simulink model "Actuator_Control"  (R2014b)
settings: Solver=FixedStepDiscrete  StartTime=0.0  StopTime=inf  FixedStep=sample_time  RelTol=1e-3
undefined symbols (not defined in the file): A1_notch_f1, A2_notch_f1, A_lpf_accel, A_lpf_dtau, B1_lpf_accel, B1_lpf_dtau, B1_notch_f1, B2_lpf_accel, B2_lpf_dtau, B2_notch_f1, gain_nodes_sea_torque, j_motor, j_segments, k_ff, K_notch_f1, k_sea, kd_loaded_sea, kd_sea_torque, kd_sea_torque_flight, kd_sea_torque_stance, kp_loaded_sea, kp_sea_torque, kp_sea_torque_flight, kp_sea_torque_stance, loaded_unloaded_sigmoid_width, loaded_unloaded_torque_threshold, max_sagittal_loaded_torque, max_sagittal_unloaded_torque, sample_time, sea_control_torque_cmd_small_threshold, sea_coulomb_friction, sea_coulomb_friction_direction_switch_sensitivity, sea_extra_sliding_friction, sea_offset_friction, stance_flight_torque_threshold
libraries: simulink x8
settings Model: BufferReuse=off  Creator=wmartin  LastModifiedBy=wmartin
settings SolverCC: EnableConcurrentExecution=on
settings DataIOCC: MaxDataPoints=1000000000  SaveFormat=StructureWithTime  SaveOutput=off  SaveTime=off
settings OptimizationCC: BlockReduction=off  OptimizeBlockIOStorage=off  BufferReuse=off  GlobalBufferReuse=off  ExpressionFolding=off  LocalBlockOutputs=off  SimCompilerOptimization=On
settings HardwareCC: ProdIntDivRoundTo=Zero  ProdEndianess=LittleEndian  ProdLongLongMode=on  ProdHWDeviceType=Generic->32-bit x86 compatible
settings ModelReferenceCC: UpdateModelReferenceTargets=AssumeUpToDate  ModelReferenceNumInstancesAllowed=Single  ModelReferenceMinAlgLoopOccurrences=on
settings RTWCC: SystemTargetFile=slrt.tlc  TemplateMakefile=slrt_default_tmf  Description=Simulink Real-Time  RTWVerbose=off  ProcessScript=slrt_make_rtw_hook  RTWCompilerOptimization=On
settings SimulinkRealTimeCC: GeneratePreprocessorConditionals=Disable all  EnableShiftOperators=on  RL32LogBufSizeModifier=100000000

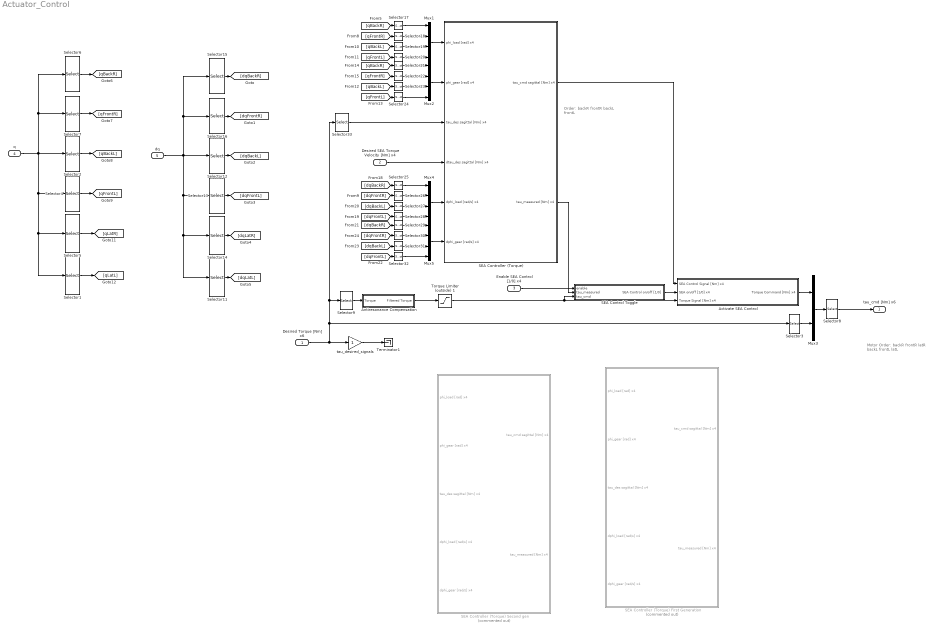
== system Actuator_Control ==
  note: Order:
      | backR
      | frontR
      | backL
      | frontL
  note: Motor Order:
      |
      | backR
      | frontR
      | latR
      | backL
      | frontL
      | latL
  Desired Torque [Nm] x6 : Inport  OutDataTypeStr=double  PortDimensions=6  SampleTime=sample_time
  Desired SEA Torque Velocity [Nm] x4 : Inport  Port=2  OutDataTypeStr=double  PortDimensions=4  SampleTime=sample_time
  Enable SEA Control [1/0] x4 : Inport  Port=3  OutDataTypeStr=boolean  PortDimensions=4  SampleTime=sample_time
  q : Inport  Port=4  OutDataTypeStr=double  PortDimensions=13  SampleTime=sample_time
  dq : Inport  Port=5  OutDataTypeStr=double  PortDimensions=13  SampleTime=sample_time
  Activate SEA Control : Subsystem
  Antiresonance Compensation : Subsystem
  Mux{1..2,4..5} (4 alike) : Mux
  Mux3 : Mux  Inputs=2
  SEA Control Toggle : Subsystem
  SEA Controller (Torque) : Subsystem
  SEA Controller (Torque) First Generation : Subsystem  Commented=on
  SEA Controller (Torque) Second gen : Subsystem  Commented=on
  Selector1 : Selector  InputPortWidth=13  Indices=[10]
  Selector11 : Selector  InputPortWidth=13  Indices=[10]
  Selector12 : Selector  InputPortWidth=13  Indices=[5 6]
  Selector13 : Selector  InputPortWidth=13  Indices=[7 8]
  Selector14 : Selector  InputPortWidth=13  Indices=[9]
  Selector15 : Selector  InputPortWidth=13  Indices=[1 2]
  Selector16 : Selector  InputPortWidth=13  Indices=[3 4]
  Selector{17..20,25..28} (8 alike) : Selector  InputPortWidth=2  Indices=[1]
  Selector2 : Selector  InputPortWidth=13  Indices=[5 6]
  Selector{21..24,29..32} (8 alike) : Selector  InputPortWidth=2  Indices=[2]
  Selector3 : Selector  InputPortWidth=6  Indices=[3 6]
  Selector33 : Selector  InputPortWidth=6  Indices=[1 2 4 5]
  Selector4 : Selector  InputPortWidth=13  Indices=[7 8]
  Selector5 : Selector  InputPortWidth=13  Indices=[9]
  Selector6 : Selector  InputPortWidth=13  Indices=[1 2]
  Selector7 : Selector  InputPortWidth=13  Indices=[3 4]
  Selector8 : Selector  InputPortWidth=6  Indices=[1 2 5 3 4 6]
  Selector9 : Selector  InputPortWidth=6  Indices=[1 2 4 5]
  Terminator1 : Terminator
  Torque Limiter (outside) 1 : Saturate  UpperLimit=max_sagittal_unloaded_torque  LowerLimit=-max_sagittal_unloaded_torque
      settings: AttributesFormatString=Hi: %<UpperLimit>\nLo: %<LowerLimit>
  tau_desired_signals : Gain  Description=xPCTag(1)=tau_cmd_signal;
  tau_cmd [Nm] x6 : Outport  OutDataTypeStr=double  PortDimensions=6  SampleTime=0  InitialOutput=[0 0 0 0 0 0]
  wires:
  Selector9/1 -> Antiresonance Compensation/1(Torque)
  SEA Controller (Torque)/2(tau_measured [Nm] x4) -> SEA Control Toggle/2(tau_measured)
  SEA Controller (Torque)/1(tau_cmd sagittal [Nm] x4) -> Activate SEA Control/1(SEA Control Signal [Nm] x4)
  Torque Limiter (outside) 1/1 -> Activate SEA Control/3(Torque Signal [Nm] x4), SEA Control Toggle/3(tau_cmd)
  Activate SEA Control/1(Torque Command [Nm] x4) -> Mux3/1
  Desired Torque [Nm] x6/1 -> Selector33/1, Selector9/1, Selector3/1, tau_desired_signals/1
  Selector8/1 -> tau_cmd [Nm] x6/1
  tau_desired_signals/1 -> Terminator1/1
  Selector5/1 -> [qLatR]
  Selector1/1 -> [qLatL]
  Selector6/1 -> [qBackR]
  Selector7/1 -> [qFrontR]
  Selector2/1 -> [qBackL]
  Selector4/1 -> [qFrontL]
  q/1 -> Selector2/1, Selector7/1, Selector6/1, Selector4/1, Selector5/1, Selector1/1
  dq/1 -> Selector11/1, Selector14/1, Selector13/1, Selector15/1, Selector16/1, Selector12/1
  Selector14/1 -> [dqLatR]
  Selector11/1 -> [dqLatL]
  Selector15/1 -> [dqBackR]
  Selector16/1 -> [dqFrontR]
  Selector12/1 -> [dqBackL]
  Selector13/1 -> [dqFrontL]
  Mux1/1 -> SEA Controller (Torque)/1(phi_load [rad] x4)
  [qBackR] -> Selector17/1
  Selector17/1 -> Mux1/1
  Selector19/1 -> Mux1/3
  Selector18/1 -> Mux1/2
  Selector20/1 -> Mux1/4
  [qFrontR] -> Selector18/1
  [qBackL] -> Selector19/1
  [qFrontL] -> Selector20/1
  Mux2/1 -> SEA Controller (Torque)/2(phi_gear [rad] x4)
  [qBackR] -> Selector21/1
  Selector21/1 -> Mux2/1
  Selector23/1 -> Mux2/3
  Selector22/1 -> Mux2/2
  Selector24/1 -> Mux2/4
  [qFrontR] -> Selector22/1
  [qBackL] -> Selector23/1
  [qFrontL] -> Selector24/1
  Mux4/1 -> SEA Controller (Torque)/5(dphi_load [rad/s] x4)
  [dqBackR] -> Selector25/1
  Selector25/1 -> Mux4/1
  Selector27/1 -> Mux4/3
  Selector26/1 -> Mux4/2
  Selector28/1 -> Mux4/4
  [dqFrontR] -> Selector26/1
  [dqBackL] -> Selector27/1
  [dqFrontL] -> Selector28/1
  Mux5/1 -> SEA Controller (Torque)/6(dphi_gear [rad/s] x4)
  [dqBackR] -> Selector29/1
  Selector29/1 -> Mux5/1
  Selector31/1 -> Mux5/3
  Selector30/1 -> Mux5/2
  Selector32/1 -> Mux5/4
  [dqFrontR] -> Selector30/1
  [dqBackL] -> Selector31/1
  [dqFrontL] -> Selector32/1
  Selector33/1 -> SEA Controller (Torque)/3(tau_des sagittal [Nm] x4)
  Selector3/1 -> Mux3/2
  Mux3/1 -> Selector8/1
  Enable SEA Control [1/0] x4/1 -> SEA Control Toggle/1(enable)
  Antiresonance Compensation/1(Filtered Torque) -> Torque Limiter (outside) 1/1
  SEA Control Toggle/1(SEA Control on/off [1/0]) -> Activate SEA Control/2("SEA on/off [1/0] x4 ")
  Desired SEA Torque Velocity [Nm] x4/1 -> SEA Controller (Torque)/4(dtau_des sagittal [Nm] x4)

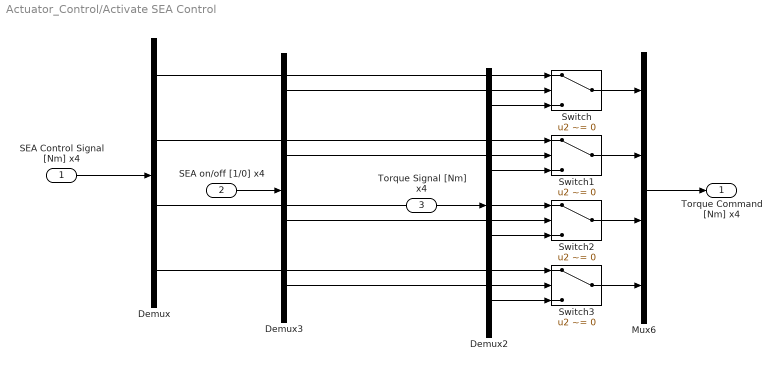
== system Actuator_Control/Activate SEA Control ==
  SEA Control Signal [Nm] x4 : Inport
  "SEA on/off [1/0] x4 " : Inport  Port=2
  Torque Signal [Nm] x4 : Inport  Port=3
  Demux : Demux
  Demux2 : Demux
  Demux3 : Demux
  Mux6 : Mux
  Switch{,1..3} (4 alike) : Switch  Criteria=u2 ~= 0
  Torque Command [Nm] x4 : Outport
  wires:
  Demux2/2 -> Switch1/3
  Demux2/1 -> Switch/3
  Demux/1 -> Switch/1
  Switch/1 -> Mux6/1
  Switch1/1 -> Mux6/2
  Switch3/1 -> Mux6/4
  Demux3/1 -> Switch/2
  Mux6/1 -> Torque Command [Nm] x4/1
  Demux3/3 -> Switch2/2
  Demux3/2 -> Switch1/2
  Demux/3 -> Switch2/1
  Switch2/1 -> Mux6/3
  Demux/4 -> Switch3/1
  Demux2/4 -> Switch3/3
  Demux3/4 -> Switch3/2
  Demux/2 -> Switch1/1
  Demux2/3 -> Switch2/3
  SEA Control Signal [Nm] x4/1 -> Demux/1
  "SEA on/off [1/0] x4 "/1 -> Demux3/1
  Torque Signal [Nm] x4/1 -> Demux2/1

== system Actuator_Control/Antiresonance Compensation ==
  Torque : Inport
  Notch Filter (Flight) : DiscreteTransferFcn  Numerator=[K_notch_f1 K_notch_f1*A1_notch_f1 K_notch_f1*A2_notch_f1]  Denominator=[1 B1_notch_f1 B2_notch_f1]  SampleTime=sample_time
  Filtered Torque : Outport
  wires:
  Torque/1 -> Notch Filter (Flight)/1
  Notch Filter (Flight)/1 -> Filtered Torque/1

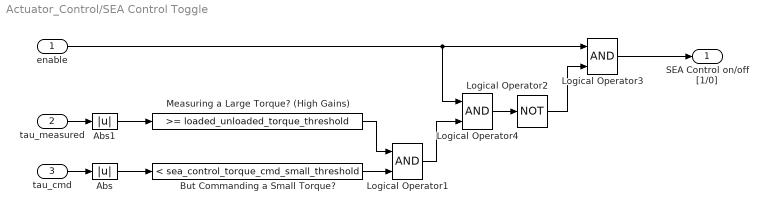
== system Actuator_Control/SEA Control Toggle ==
  enable : Inport
  tau_measured : Inport  Port=2
  tau_cmd : Inport  Port=3
  Abs : Abs
  Abs1 : Abs
  But Commanding a Small Torque? : simulink/Logic and Bit Operations/Compare To Constant  relop=<  const=sea_control_torque_cmd_small_threshold  OutDataTypeStr=boolean
  Logical Operator1 : Logic  AllPortsSameDT=off  OutDataTypeStr=boolean
  Logical Operator2 : Logic  Operator=NOT  AllPortsSameDT=off  OutDataTypeStr=boolean
  Logical Operator3 : Logic  AllPortsSameDT=off  OutDataTypeStr=boolean
  Logical Operator4 : Logic  AllPortsSameDT=off  OutDataTypeStr=boolean
  Measuring a Large Torque? (High Gains) : simulink/Logic and Bit Operations/Compare To Constant  relop=>=  const=loaded_unloaded_torque_threshold  OutDataTypeStr=boolean
  SEA Control on/off [1/0] : Outport
  wires:
  But Commanding a Small Torque?/1 -> Logical Operator1/2
  Logical Operator1/1 -> Logical Operator4/2
  tau_cmd/1 -> Abs/1
  Abs/1 -> But Commanding a Small Torque?/1
  tau_measured/1 -> Abs1/1
  Abs1/1 -> Measuring a Large Torque? (High Gains)/1
  Logical Operator3/1 -> SEA Control on/off [1/0]/1
  Logical Operator2/1 -> Logical Operator3/2
  Logical Operator4/1 -> Logical Operator2/1
  enable/1 -> Logical Operator4/1, Logical Operator3/1
  Measuring a Large Torque? (High Gains)/1 -> Logical Operator1/1

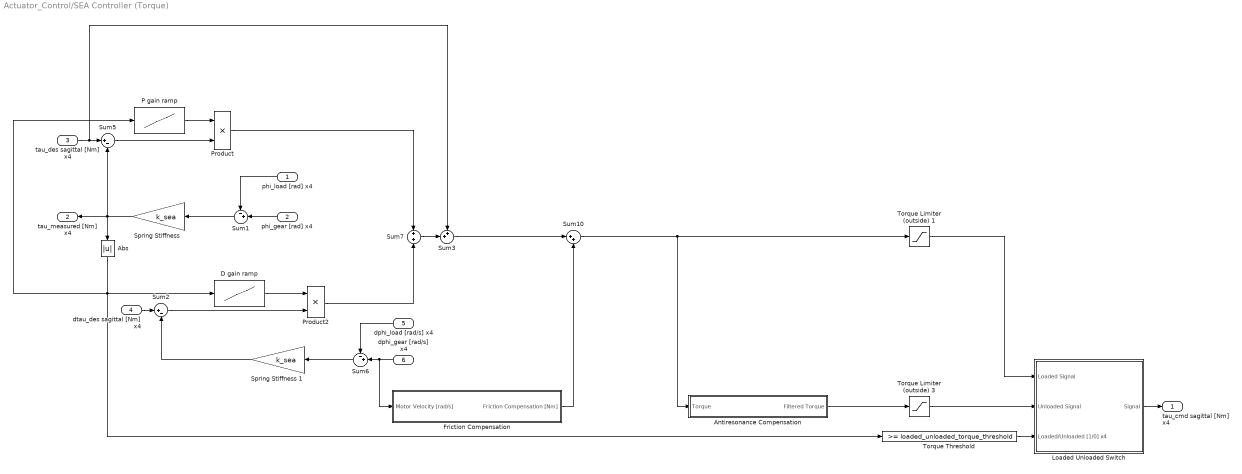
== system Actuator_Control/SEA Controller (Torque) ==
  phi_load [rad] x4 : Inport
  phi_gear [rad] x4 : Inport  Port=2
  tau_des sagittal [Nm] x4 : Inport  Port=3
  dtau_des sagittal [Nm] x4 : Inport  Port=4
  dphi_load [rad/s] x4 : Inport  Port=5
  dphi_gear [rad/s] x4 : Inport  Port=6
  Abs : Abs
  Antiresonance Compensation : Subsystem
  D gain ramp : Lookup_n-D  NumberOfTableDimensions=1  BreakpointsForDimension1=gain_nodes_sea_torque  Table=kd_sea_torque  InternalRulePriority=Speed  RndMeth=Simplest  InputSameDT=on
  Friction Compensation : Subsystem
  Loaded Unloaded Switch : Subsystem
  P gain ramp : Lookup_n-D  NumberOfTableDimensions=1  BreakpointsForDimension1=gain_nodes_sea_torque  Table=kp_sea_torque  InternalRulePriority=Speed  RndMeth=Simplest  InputSameDT=on
  Product : Product  SampleTime=sample_time  RndMeth=Zero
  Product2 : Product  RndMeth=Zero
  Spring Stiffness : Gain  Gain=k_sea
  Spring Stiffness 1 : Gain  Gain=k_sea
  Sum1 : Sum  Inputs=-+|
  Sum10 : Sum  Inputs=|++
  Sum2 : Sum  Inputs=|+-
  Sum3 : Sum  Inputs=++|
  Sum5 : Sum  Inputs=|+-
  Sum6 : Sum  Inputs=-+|
  Sum7 : Sum  Inputs=+|+
  Torque Limiter (outside) 1 : Saturate  UpperLimit=max_sagittal_loaded_torque  LowerLimit=-max_sagittal_loaded_torque
      settings: AttributesFormatString=Hi: %<UpperLimit>\nLo: %<LowerLimit>
  Torque Limiter (outside) 3 : Saturate  UpperLimit=max_sagittal_unloaded_torque  LowerLimit=-max_sagittal_unloaded_torque
      settings: AttributesFormatString=Hi: %<UpperLimit>\nLo: %<LowerLimit>
  Torque Threshold : simulink/Logic and Bit Operations/Compare To Constant  relop=>=  const=loaded_unloaded_torque_threshold  OutDataTypeStr=boolean
  tau_cmd sagittal [Nm] x4 : Outport
  tau_measured [Nm] x4 : Outport  Port=2
  wires:
  Product2/1 -> Sum7/2
  D gain ramp/1 -> Product2/1
  Sum2/1 -> Product2/2
  Sum5/1 -> Product/2
  dphi_gear [rad/s] x4/1 -> Friction Compensation/1(Motor Velocity [rad/s]), Sum6/2
  dphi_load [rad/s] x4/1 -> Sum6/1
  Spring Stiffness 1/1 -> Sum2/2
  Sum6/1 -> Spring Stiffness 1/1
  dtau_des sagittal [Nm] x4/1 -> Sum2/1
  tau_des sagittal [Nm] x4/1 -> Sum5/1, Sum3/1
  phi_gear [rad] x4/1 -> Sum1/2
  phi_load [rad] x4/1 -> Sum1/1
  Sum1/1 -> Spring Stiffness/1
  Spring Stiffness/1 -> Sum5/2, Abs/1, tau_measured [Nm] x4/1
  Sum10/1 -> Antiresonance Compensation/1(Torque), Torque Limiter (outside) 1/1
  P gain ramp/1 -> Product/1
  Product/1 -> Sum7/1
  Sum7/1 -> Sum3/2
  Torque Limiter (outside) 1/1 -> Loaded Unloaded Switch/1(Loaded Signal)
  Torque Limiter (outside) 3/1 -> Loaded Unloaded Switch/2(Unloaded Signal)
  Antiresonance Compensation/1(Filtered Torque) -> Torque Limiter (outside) 3/1
  Friction Compensation/1(Friction Compensation [Nm]) -> Sum10/2
  Loaded Unloaded Switch/1(Signal) -> tau_cmd sagittal [Nm] x4/1
  Torque Threshold/1 -> Loaded Unloaded Switch/3(Loaded/Unloaded [1/0] x4)
  Abs/1 -> D gain ramp/1, P gain ramp/1, Torque Threshold/1
  Sum3/1 -> Sum10/1

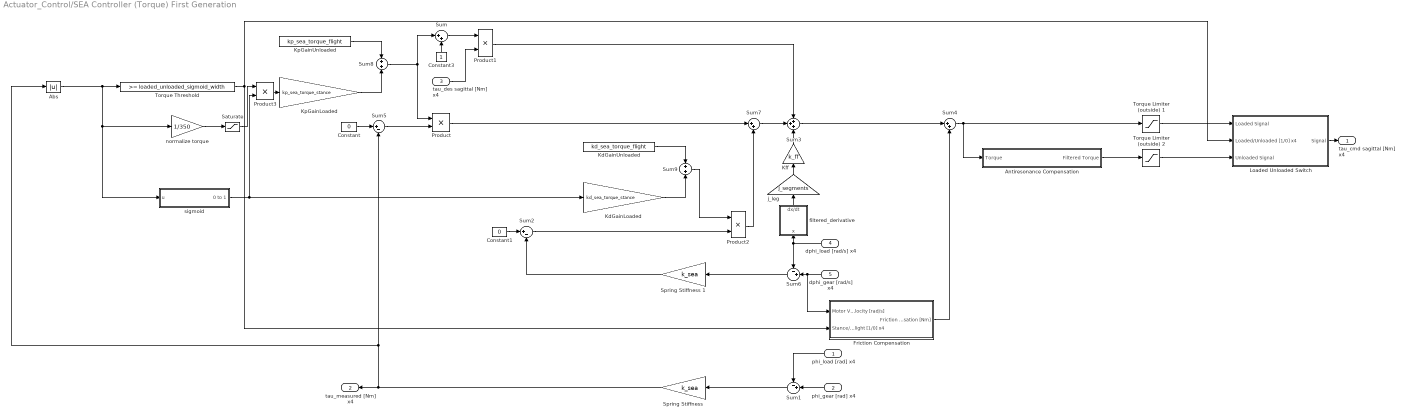
== system Actuator_Control/SEA Controller (Torque) First Generation ==
  phi_load [rad] x4 : Inport
  phi_gear [rad] x4 : Inport  Port=2
  tau_des sagittal [Nm] x4 : Inport  Port=3
  dphi_load [rad/s] x4 : Inport  Port=4
  dphi_gear [rad/s] x4 : Inport  Port=5
  Abs : Abs
  Antiresonance Compensation : Subsystem
  Constant : Constant  Value=0
  Constant1 : Constant  Value=0
  Constant3 : Constant
  Friction Compensation : Subsystem
  KdGainLoaded : Gain  Description=xPCTag(1)=kd_sea_torque;  Gain=kd_sea_torque_stance
  KdGainUnloaded : Constant  Value=kd_sea_torque_flight  SampleTime=sample_time
  Kff : Gain  Gain=k_ff
  KpGainLoaded : Gain  Description=xPCTag(1)=kd_sea_torque;  Gain=kp_sea_torque_stance
  KpGainUnloaded : Constant  Value=kp_sea_torque_flight  SampleTime=sample_time
  Loaded Unloaded Switch : Subsystem
  Product : Product  SampleTime=sample_time  RndMeth=Zero
  Product1 : Product  RndMeth=Zero
  Product2 : Product  RndMeth=Zero
  Product3 : Product  SampleTime=sample_time  RndMeth=Zero
  Saturate : Saturate  UpperLimit=1  LowerLimit=0
      settings: AttributesFormatString=Hi: %<UpperLimit>\nLo: %<LowerLimit>
  Spring Stiffness : Gain  Gain=k_sea
  Spring Stiffness 1 : Gain  Gain=k_sea
  Sum : Sum  Inputs=|++  SampleTime=sample_time
  Sum1 : Sum  Inputs=-+|
  Sum2 : Sum  Inputs=|+-
  Sum3 : Sum  Inputs=+++
  Sum4 : Sum  Inputs=|++
  Sum5 : Sum  Inputs=|+-
  Sum6 : Sum  Inputs=-+|
  Sum7 : Sum  Inputs=|++
  Sum8 : Sum  Inputs=+|+  SampleTime=sample_time
  Sum9 : Sum  Inputs=+|+  SampleTime=sample_time
  Torque Limiter (outside) 1 : Saturate  UpperLimit=max_sagittal_loaded_torque  LowerLimit=-max_sagittal_loaded_torque
      settings: AttributesFormatString=Hi: %<UpperLimit>\nLo: %<LowerLimit>
  Torque Limiter (outside) 2 : Saturate  UpperLimit=max_sagittal_unloaded_torque  LowerLimit=-max_sagittal_unloaded_torque
      settings: AttributesFormatString=Hi: %<UpperLimit>\nLo: %<LowerLimit>
  Torque Threshold : simulink/Logic and Bit Operations/Compare To Constant  relop=>=  const=loaded_unloaded_sigmoid_width  OutDataTypeStr=boolean
  filtered_derivative : Subsystem
  j_leg : Gain  Description=xPCTag(1)=kd_sea_torque;  Gain=j_segments
  normalize torque : Gain  Description=xPCTag(1)=kd_sea_torque;  Gain=1/350
  sigmoid : Subsystem
  tau_cmd sagittal [Nm] x4 : Outport
  tau_measured [Nm] x4 : Outport  Port=2
  wires:
  Product2/1 -> Sum7/2
  Sum9/1 -> Product2/1
  Sum2/1 -> Product2/2
  sigmoid/1(0 to 1) -> KdGainLoaded/1, Product3/2
  KdGainLoaded/1 -> Sum9/2
  KdGainUnloaded/1 -> Sum9/1
  KpGainLoaded/1 -> Sum8/2
  KpGainUnloaded/1 -> Sum8/1
  Loaded Unloaded Switch/1(Signal) -> tau_cmd sagittal [Nm] x4/1
  Torque Limiter (outside) 2/1 -> Loaded Unloaded Switch/3(Unloaded Signal)
  Friction Compensation/1(Friction Compensation [Nm]) -> Sum4/2
  tau_des sagittal [Nm] x4/1 -> Product1/2
  Kff/1 -> Sum3/3
  Torque Limiter (outside) 1/1 -> Loaded Unloaded Switch/1(Loaded Signal)
  j_leg/1 -> Kff/1
  filtered_derivative/1(dx/dt) -> j_leg/1
  Sum/1 -> Product1/1
  Constant3/1 -> Sum/2
  Product/1 -> Sum7/1
  Sum5/1 -> Product/2
  dphi_gear [rad/s] x4/1 -> Sum6/2, Friction Compensation/1(Motor Velocity [rad/s])
  dphi_load [rad/s] x4/1 -> filtered_derivative/1(x), Sum6/1
  Spring Stiffness 1/1 -> Sum2/2
  Sum6/1 -> Spring Stiffness 1/1
  Constant1/1 -> Sum2/1
  Constant/1 -> Sum5/1
  phi_gear [rad] x4/1 -> Sum1/2
  phi_load [rad] x4/1 -> Sum1/1
  Sum1/1 -> Spring Stiffness/1
  Torque Threshold/1 -> Friction Compensation/2(Stance/Flight [1/0] x4), Loaded Unloaded Switch/2(Loaded/Unloaded [1/0] x4)
  Spring Stiffness/1 -> Sum5/2, Abs/1, tau_measured [Nm] x4/1
  Sum8/1 -> Product/1, Sum/1
  Abs/1 -> sigmoid/1(u), normalize torque/1, Torque Threshold/1
  Sum4/1 -> Torque Limiter (outside) 1/1, Antiresonance Compensation/1(Torque)
  Product1/1 -> Sum3/1
  Sum7/1 -> Sum3/2
  Sum3/1 -> Sum4/1
  Antiresonance Compensation/1(Filtered Torque) -> Torque Limiter (outside) 2/1
  normalize torque/1 -> Saturate/1
  Product3/1 -> KpGainLoaded/1
  Saturate/1 -> Product3/1

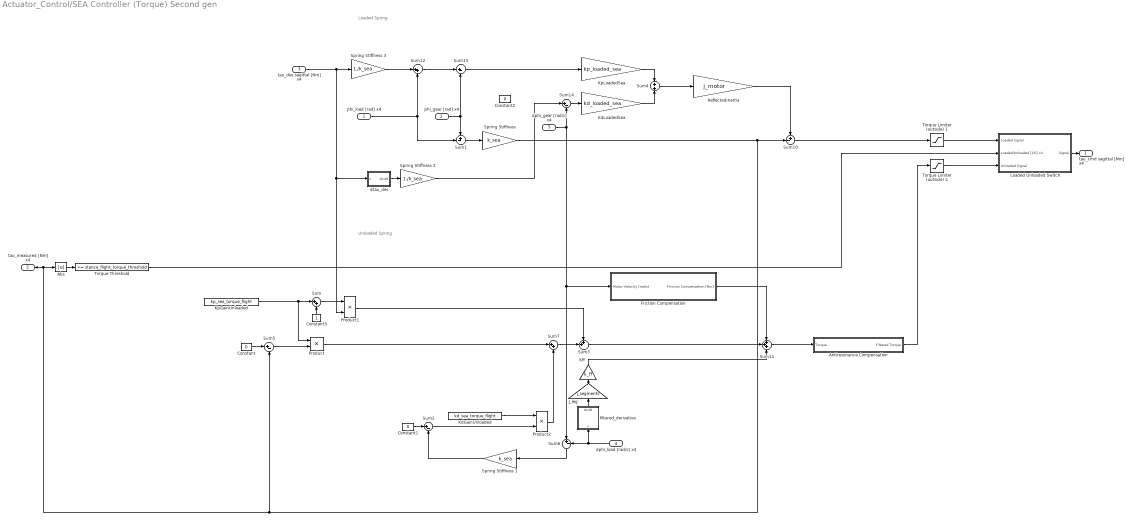
== system Actuator_Control/SEA Controller (Torque) Second gen ==
  note: Loaded Spring
  note: Unloaded Spring
  phi_load [rad] x4 : Inport
  phi_gear [rad] x4 : Inport  Port=2
  tau_des sagittal [Nm] x4 : Inport  Port=3
  dphi_load [rad/s] x4 : Inport  Port=4
  dphi_gear [rad/s] x4 : Inport  Port=5
  Abs : Abs
  Antiresonance Compensation : Subsystem
  Constant : Constant  Value=0
  Constant1 : Constant  Value=0
  Constant2 : Constant  Value=0
  Constant3 : Constant
  Friction Compensation : Subsystem
  KdGainUnloaded : Constant  Value=kd_sea_torque_flight  SampleTime=sample_time
  KdLoadedSea : Gain  Description=xPCTag(1)=kd_sea_torque;  Gain=kd_loaded_sea
  Kff : Gain  Gain=k_ff
  KpGainUnloaded : Constant  Value=kp_sea_torque_flight  SampleTime=sample_time
  KpLoadedSea : Gain  Description=xPCTag(1)=kd_sea_torque;  Gain=kp_loaded_sea
  Loaded Unloaded Switch : Subsystem
  Product : Product  SampleTime=sample_time  RndMeth=Zero
  Product1 : Product  RndMeth=Zero
  Product2 : Product  RndMeth=Zero
  ReflectedInertia : Gain  Description=xPCTag(1)=kd_sea_torque;  Gain=j_motor
  Spring Stiffness : Gain  Gain=k_sea
  Spring Stiffness 1 : Gain  Gain=k_sea
  Spring Stiffness 2 : Gain  Gain=1./k_sea
  Spring Stiffness 3 : Gain  Gain=1./k_sea
  Sum : Sum  Inputs=|++  SampleTime=sample_time
  Sum1 : Sum  Inputs=+-|
  Sum10 : Sum  Inputs=+-|
  Sum11 : Sum  Inputs=+++
  Sum12 : Sum  Inputs=|++
  Sum{2,5..6,13..14} (5 alike) : Sum  Inputs=|+-
  Sum3 : Sum  Inputs=++|
  Sum4 : Sum  Inputs=+|+  SampleTime=sample_time
  Sum7 : Sum  Inputs=|++
  Torque Limiter (outside) 1 : Saturate  UpperLimit=max_sagittal_loaded_torque  LowerLimit=-max_sagittal_loaded_torque
      settings: AttributesFormatString=Hi: %<UpperLimit>\nLo: %<LowerLimit>
  Torque Limiter (outside) 2 : Saturate  UpperLimit=max_sagittal_unloaded_torque  LowerLimit=-max_sagittal_unloaded_torque
      settings: AttributesFormatString=Hi: %<UpperLimit>\nLo: %<LowerLimit>
  Torque Threshold : simulink/Logic and Bit Operations/Compare To Constant  relop=>=  const=stance_flight_torque_threshold  OutDataTypeStr=boolean
  dtau_des : Subsystem
  filtered_derivative : Subsystem
  j_leg : Gain  Description=xPCTag(1)=kd_sea_torque;  Gain=j_segments
  tau_cmd sagittal [Nm] x4 : Outport
  tau_measured [Nm] x4 : Outport  Port=2
  wires:
  Antiresonance Compensation/1(Filtered Torque) -> Torque Limiter (outside) 2/1
  Sum7/1 -> Sum3/2
  Product1/1 -> Sum3/1
  Sum3/1 -> Sum11/2
  Abs/1 -> Torque Threshold/1
  KpGainUnloaded/1 -> Product/1, Sum/1
  Torque Threshold/1 -> Loaded Unloaded Switch/2(Loaded/Unloaded [1/0] x4)
  Sum1/1 -> Spring Stiffness/1
  phi_load [rad] x4/1 -> Sum1/2, Sum12/2
  phi_gear [rad] x4/1 -> Sum1/1, Sum13/2
  Constant/1 -> Sum5/1
  Constant1/1 -> Sum2/1
  Sum6/1 -> Spring Stiffness 1/1
  Spring Stiffness 1/1 -> Sum2/2
  dphi_load [rad/s] x4/1 -> filtered_derivative/1(x), Sum6/2
  dphi_gear [rad/s] x4/1 -> Sum14/2, Sum6/1, Friction Compensation/1(Motor Velocity [rad/s])
  Sum5/1 -> Product/2
  Product/1 -> Sum7/1
  Constant3/1 -> Sum/2
  Sum/1 -> Product1/1
  filtered_derivative/1(dx/dt) -> j_leg/1
  j_leg/1 -> Kff/1
  Torque Limiter (outside) 1/1 -> Loaded Unloaded Switch/1(Loaded Signal)
  Kff/1 -> Sum11/3
  tau_des sagittal [Nm] x4/1 -> Spring Stiffness 3/1, Product1/2, dtau_des/1(x)
  Torque Limiter (outside) 2/1 -> Loaded Unloaded Switch/3(Unloaded Signal)
  Loaded Unloaded Switch/1(Signal) -> tau_cmd sagittal [Nm] x4/1
  Sum2/1 -> Product2/2
  KdGainUnloaded/1 -> Product2/1
  Product2/1 -> Sum7/2
  Spring Stiffness/1 -> Sum10/2, Abs/1, tau_measured [Nm] x4/1, Sum5/2
  Sum10/1 -> Torque Limiter (outside) 1/1
  Sum11/1 -> Antiresonance Compensation/1(Torque)
  Friction Compensation/1(Friction Compensation [Nm]) -> Sum11/1
  ReflectedInertia/1 -> Sum10/1
  Sum4/1 -> ReflectedInertia/1
  KdLoadedSea/1 -> Sum4/2
  KpLoadedSea/1 -> Sum4/1
  Spring Stiffness 3/1 -> Sum12/1
  Sum12/1 -> Sum13/1
  Spring Stiffness 2/1 -> Sum14/1
  Sum14/1 -> KdLoadedSea/1
  Sum13/1 -> KpLoadedSea/1
  dtau_des/1(dx/dt) -> Spring Stiffness 2/1

== system Actuator_Control/SEA Controller (Torque)/Antiresonance Compensation ==
  Torque : Inport
  Notch Filter (Flight) : DiscreteTransferFcn  Numerator=[K_notch_f1 K_notch_f1*A1_notch_f1 K_notch_f1*A2_notch_f1]  Denominator=[1 B1_notch_f1 B2_notch_f1]  SampleTime=sample_time
  Filtered Torque : Outport
  wires:
  Notch Filter (Flight)/1 -> Filtered Torque/1
  Torque/1 -> Notch Filter (Flight)/1

== system Actuator_Control/SEA Controller (Torque)/Friction Compensation ==
  Motor Velocity [rad/s] : Inport
  Gain2 : Gain  Gain=sea_coulomb_friction_direction_switch_sensitivity
  KdGain2 : Gain  Description=xPCTag(1)=kd_sea_torque;  Gain=sea_coulomb_friction
  Trigonometric Function : Trigonometry  Operator=tanh
  Friction Compensation [Nm] : Outport
  wires:
  Trigonometric Function/1 -> KdGain2/1
  Gain2/1 -> Trigonometric Function/1
  Motor Velocity [rad/s]/1 -> Gain2/1
  KdGain2/1 -> Friction Compensation [Nm]/1

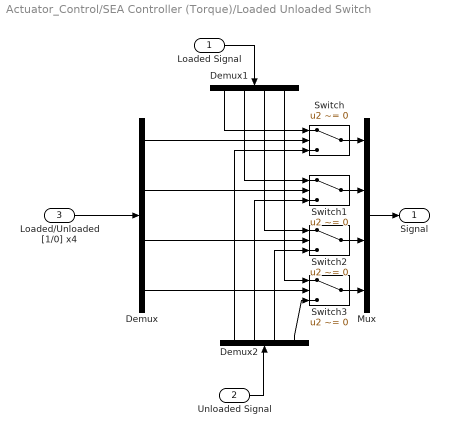
== system Actuator_Control/SEA Controller (Torque)/Loaded Unloaded Switch ==
  Loaded Signal : Inport
  Unloaded Signal : Inport  Port=2
  Loaded/Unloaded [1/0] x4 : Inport  Port=3
  Demux : Demux
  Demux1 : Demux
  Demux2 : Demux
  Mux : Mux
  Switch{,1..3} (4 alike) : Switch  Criteria=u2 ~= 0
  Signal : Outport
  wires:
  Demux2/1 -> Switch/3
  Demux2/2 -> Switch1/3
  Demux2/3 -> Switch2/3
  Demux2/4 -> Switch3/3
  Unloaded Signal/1 -> Demux2/1
  Demux1/4 -> Switch3/1
  Demux1/3 -> Switch2/1
  Demux1/2 -> Switch1/1
  Demux1/1 -> Switch/1
  Loaded Signal/1 -> Demux1/1
  Demux/1 -> Switch/2
  Switch/1 -> Mux/1
  Mux/1 -> Signal/1
  Loaded/Unloaded [1/0] x4/1 -> Demux/1
  Switch3/1 -> Mux/4
  Switch2/1 -> Mux/3
  Switch1/1 -> Mux/2
  Demux/2 -> Switch1/2
  Demux/3 -> Switch2/2
  Demux/4 -> Switch3/2

== system Actuator_Control/SEA Controller (Torque) First Generation/Antiresonance Compensation ==
  Torque : Inport
  Notch Filter (Flight) : DiscreteTransferFcn  Numerator=[K_notch_f1 K_notch_f1*A1_notch_f1 K_notch_f1*A2_notch_f1]  Denominator=[1 B1_notch_f1 B2_notch_f1]  SampleTime=sample_time
  Filtered Torque : Outport
  wires:
  Notch Filter (Flight)/1 -> Filtered Torque/1
  Torque/1 -> Notch Filter (Flight)/1

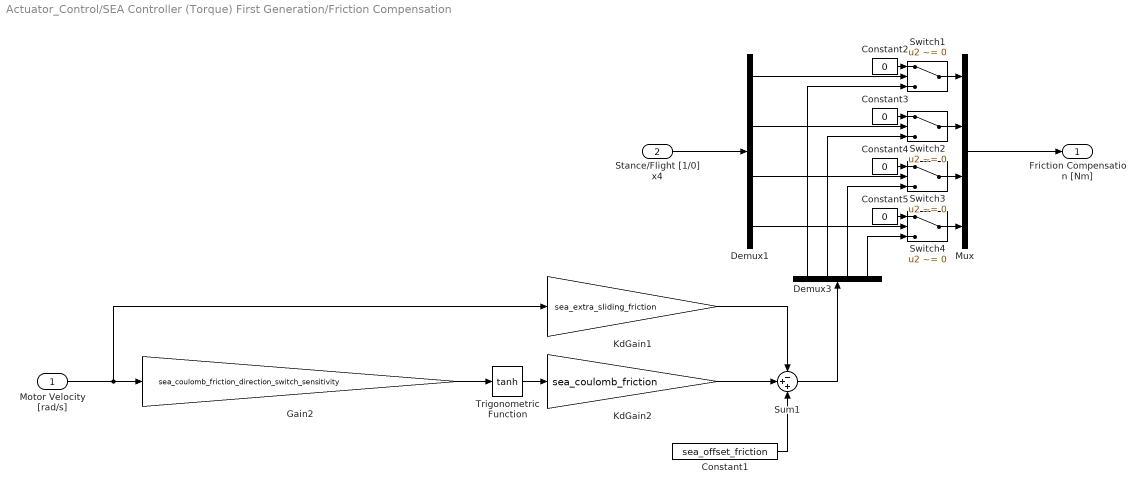
== system Actuator_Control/SEA Controller (Torque) First Generation/Friction Compensation ==
  Motor Velocity [rad/s] : Inport
  Stance/Flight [1/0] x4 : Inport  Port=2
  Constant1 : Constant  Value=sea_offset_friction
  Constant{2..5} (4 alike) : Constant  Value=0
  Demux1 : Demux
  Demux3 : Demux
  Gain2 : Gain  Gain=sea_coulomb_friction_direction_switch_sensitivity
  KdGain1 : Gain  Description=xPCTag(1)=kd_sea_torque;  Gain=sea_extra_sliding_friction
  KdGain2 : Gain  Description=xPCTag(1)=kd_sea_torque;  Gain=sea_coulomb_friction
  Mux : Mux
  Sum1 : Sum  Inputs=-++
  Switch{1..4} (4 alike) : Switch  Criteria=u2 ~= 0
  Trigonometric Function : Trigonometry  Operator=tanh
  Friction Compensation [Nm] : Outport
  wires:
  KdGain1/1 -> Sum1/1
  Mux/1 -> Friction Compensation [Nm]/1
  Trigonometric Function/1 -> KdGain2/1
  Gain2/1 -> Trigonometric Function/1
  Motor Velocity [rad/s]/1 -> Gain2/1, KdGain1/1
  KdGain2/1 -> Sum1/2
  Constant1/1 -> Sum1/3
  Demux1/4 -> Switch4/2
  Demux1/3 -> Switch3/2
  Demux1/2 -> Switch2/2
  Switch2/1 -> Mux/2
  Switch3/1 -> Mux/3
  Switch4/1 -> Mux/4
  Switch1/1 -> Mux/1
  Demux1/1 -> Switch1/2
  Demux3/4 -> Switch4/3
  Demux3/3 -> Switch3/3
  Demux3/2 -> Switch2/3
  Demux3/1 -> Switch1/3
  Stance/Flight [1/0] x4/1 -> Demux1/1
  Constant2/1 -> Switch1/1
  Constant3/1 -> Switch2/1
  Constant4/1 -> Switch3/1
  Constant5/1 -> Switch4/1
  Sum1/1 -> Demux3/1

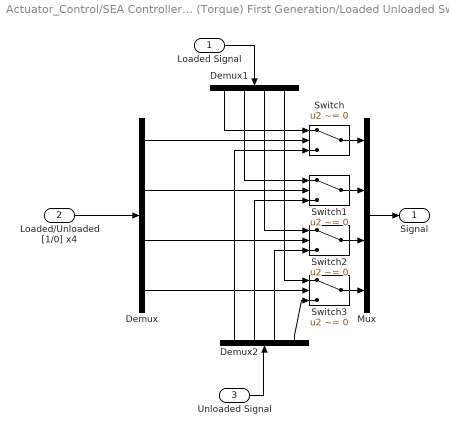
== system Actuator_Control/SEA Controller (Torque) First Generation/Loaded Unloaded Switch ==
  Loaded Signal : Inport
  Loaded/Unloaded [1/0] x4 : Inport  Port=2
  Unloaded Signal : Inport  Port=3
  Demux : Demux
  Demux1 : Demux
  Demux2 : Demux
  Mux : Mux
  Switch{,1..3} (4 alike) : Switch  Criteria=u2 ~= 0
  Signal : Outport
  wires:
  Demux2/1 -> Switch/3
  Demux2/2 -> Switch1/3
  Demux2/3 -> Switch2/3
  Demux2/4 -> Switch3/3
  Unloaded Signal/1 -> Demux2/1
  Demux1/4 -> Switch3/1
  Demux1/3 -> Switch2/1
  Demux1/2 -> Switch1/1
  Demux1/1 -> Switch/1
  Loaded Signal/1 -> Demux1/1
  Demux/1 -> Switch/2
  Switch/1 -> Mux/1
  Mux/1 -> Signal/1
  Loaded/Unloaded [1/0] x4/1 -> Demux/1
  Switch3/1 -> Mux/4
  Switch2/1 -> Mux/3
  Switch1/1 -> Mux/2
  Demux/2 -> Switch1/2
  Demux/3 -> Switch2/2
  Demux/4 -> Switch3/2

== system Actuator_Control/SEA Controller (Torque) First Generation/filtered_derivative ==
  x : Inport
  Gain1 : Gain  Gain=1/sample_time
  difference : simulink/Discrete/Difference  ICPrevInput=0.0  InputProcessing=Inherited  OutMin=[]  OutMax=[]  OutDataType=fixdt(1, 16)  OutScaling=2^-10  DoSatur=off
  two_pole_filter : DiscreteTransferFcn  Numerator=[A_lpf_accel 0 0]  Denominator=[1 B1_lpf_accel B2_lpf_accel]  SampleTime=sample_time
  dx/dt : Outport
  wires:
  Gain1/1 -> difference/1
  difference/1 -> two_pole_filter/1
  x/1 -> Gain1/1
  two_pole_filter/1 -> dx/dt/1

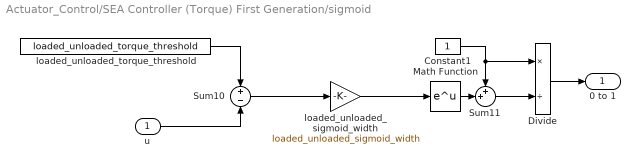
== system Actuator_Control/SEA Controller (Torque) First Generation/sigmoid ==
  u : Inport
  Constant1 : Constant
  Divide : Product  Inputs=*/
  Math Function : Math  SaturateOnIntegerOverflow=on
  Sum10 : Sum  Inputs=+|-  SampleTime=sample_time
  Sum11 : Sum  Inputs=++|  SampleTime=sample_time
  loaded_unloaded_sigmoid_width : Gain  Gain=loaded_unloaded_sigmoid_width
  loaded_unloaded_torque_threshold : Constant  Value=loaded_unloaded_torque_threshold  SampleTime=sample_time
  0 to 1 : Outport
  wires:
  Sum11/1 -> Divide/2
  u/1 -> Sum10/2
  Math Function/1 -> Sum11/2
  Constant1/1 -> Divide/1, Sum11/1
  loaded_unloaded_torque_threshold/1 -> Sum10/1
  Sum10/1 -> loaded_unloaded_sigmoid_width/1
  Divide/1 -> 0 to 1/1
  loaded_unloaded_sigmoid_width/1 -> Math Function/1

== system Actuator_Control/SEA Controller (Torque) Second gen/Antiresonance Compensation ==
  Torque : Inport
  Notch Filter (Flight) : DiscreteTransferFcn  Numerator=[K_notch_f1 K_notch_f1*A1_notch_f1 K_notch_f1*A2_notch_f1]  Denominator=[1 B1_notch_f1 B2_notch_f1]  SampleTime=sample_time
  Filtered Torque : Outport
  wires:
  Torque/1 -> Notch Filter (Flight)/1
  Notch Filter (Flight)/1 -> Filtered Torque/1

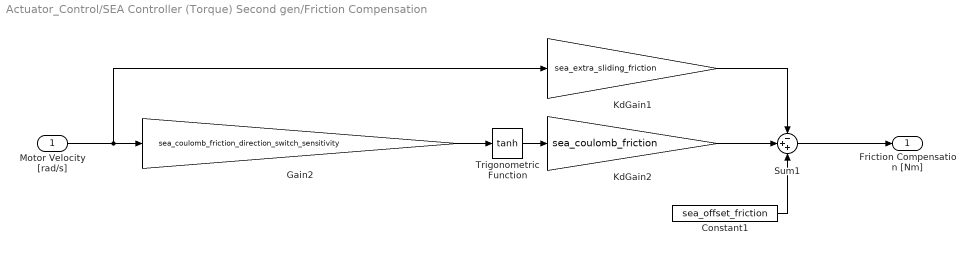
== system Actuator_Control/SEA Controller (Torque) Second gen/Friction Compensation ==
  Motor Velocity [rad/s] : Inport
  Constant1 : Constant  Value=sea_offset_friction
  Gain2 : Gain  Gain=sea_coulomb_friction_direction_switch_sensitivity
  KdGain1 : Gain  Description=xPCTag(1)=kd_sea_torque;  Gain=sea_extra_sliding_friction
  KdGain2 : Gain  Description=xPCTag(1)=kd_sea_torque;  Gain=sea_coulomb_friction
  Sum1 : Sum  Inputs=-++
  Trigonometric Function : Trigonometry  Operator=tanh
  Friction Compensation [Nm] : Outport
  wires:
  Constant1/1 -> Sum1/3
  KdGain2/1 -> Sum1/2
  Motor Velocity [rad/s]/1 -> KdGain1/1, Gain2/1
  Gain2/1 -> Trigonometric Function/1
  Trigonometric Function/1 -> KdGain2/1
  KdGain1/1 -> Sum1/1
  Sum1/1 -> Friction Compensation [Nm]/1

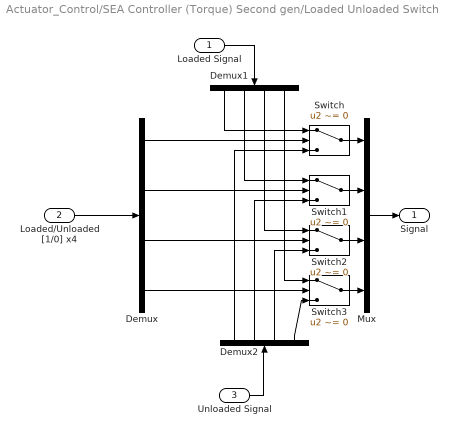
== system Actuator_Control/SEA Controller (Torque) Second gen/Loaded Unloaded Switch ==
  Loaded Signal : Inport
  Loaded/Unloaded [1/0] x4 : Inport  Port=2
  Unloaded Signal : Inport  Port=3
  Demux : Demux
  Demux1 : Demux
  Demux2 : Demux
  Mux : Mux
  Switch{,1..3} (4 alike) : Switch  Criteria=u2 ~= 0
  Signal : Outport
  wires:
  Demux/4 -> Switch3/2
  Demux/3 -> Switch2/2
  Demux/2 -> Switch1/2
  Switch1/1 -> Mux/2
  Switch2/1 -> Mux/3
  Switch3/1 -> Mux/4
  Loaded/Unloaded [1/0] x4/1 -> Demux/1
  Mux/1 -> Signal/1
  Switch/1 -> Mux/1
  Demux/1 -> Switch/2
  Loaded Signal/1 -> Demux1/1
  Demux1/1 -> Switch/1
  Demux1/2 -> Switch1/1
  Demux1/3 -> Switch2/1
  Demux1/4 -> Switch3/1
  Unloaded Signal/1 -> Demux2/1
  Demux2/4 -> Switch3/3
  Demux2/3 -> Switch2/3
  Demux2/2 -> Switch1/3
  Demux2/1 -> Switch/3

== system Actuator_Control/SEA Controller (Torque) Second gen/dtau_des ==
  x : Inport
  Gain1 : Gain  Gain=1/sample_time
  difference : simulink/Discrete/Difference  ICPrevInput=0.0  InputProcessing=Inherited  OutMin=[]  OutMax=[]  OutDataType=fixdt(1, 16)  OutScaling=2^-10  DoSatur=off
  two_pole_filter : DiscreteTransferFcn  Numerator=[A_lpf_dtau 0 0]  Denominator=[1 B1_lpf_dtau B2_lpf_dtau]  SampleTime=sample_time
  dx/dt : Outport
  wires:
  Gain1/1 -> difference/1
  difference/1 -> two_pole_filter/1
  x/1 -> Gain1/1
  two_pole_filter/1 -> dx/dt/1

== system Actuator_Control/SEA Controller (Torque) Second gen/filtered_derivative ==
  x : Inport
  Gain1 : Gain  Gain=1/sample_time
  difference : simulink/Discrete/Difference  ICPrevInput=0.0  InputProcessing=Inherited  OutMin=[]  OutMax=[]  OutDataType=fixdt(1, 16)  OutScaling=2^-10  DoSatur=off
  two_pole_filter : DiscreteTransferFcn  Numerator=[A_lpf_accel 0 0]  Denominator=[1 B1_lpf_accel B2_lpf_accel]  SampleTime=sample_time
  dx/dt : Outport
  wires:
  two_pole_filter/1 -> dx/dt/1
  x/1 -> Gain1/1
  difference/1 -> two_pole_filter/1
  Gain1/1 -> difference/1
